simulink model "my_dom_model"  (R2018a)
settings: Solver=VariableStepAuto  StartTime=0.0  StopTime=10000  RelTol=1e-3
values from neighbouring files (symbols this model uses):
  c_p = 1000    [leveled_NL.m]    (also in leveled_state_space.m; leveled_transmitancja.m; my_dom.m; my_dom_state_space_script.m)
  C_vp = c_p*ro_p*V_p    (= 120000)    [leveled_NL.m]    (also in leveled_state_space.m; leveled_transmitancja.m; my_dom.m; my_dom_state_space_script.m)
  C_vw = c_p*ro_p*V_w    (= 1200000)    [leveled_NL.m]    (also in leveled_state_space.m; leveled_transmitancja.m; my_dom.m; my_dom_state_space_script.m)
  d_f_p = 0.2    [leveled_NL.m]    (also in leveled_state_space.m = 0; leveled_transmitancja.m = 0; my_dom.m; my_dom_state_space_script.m = 0)
  d_T_z = 0    [leveled_NL.m]    (also in leveled_state_space.m; leveled_transmitancja.m; my_dom.m; my_dom_state_space_script.m)
  d_T_zew = 0    [leveled_NL.m]    (also in leveled_state_space.m = 2; leveled_transmitancja.m = 2; my_dom.m; my_dom_state_space_script.m = 5)
  f_p1 = f_pN-0.35    (= 0.65)    [leveled_NL.m]    (also in leveled_state_space.m = 1; leveled_transmitancja.m = 1; my_dom.m = 1.25; my_dom_statyczne.m = 0.1:0.1:25)
  K_1 = K_matrix(1,1)    [leveled_NL.m]    (also in leveled_state_space.m; leveled_transmitancja.m; my_dom.m; my_dom_state_space_script.m)
  K_p = p*K_w    [leveled_NL.m]    (also in leveled_state_space.m; leveled_transmitancja.m; my_dom.m; my_dom_state_space_script.m)
  K_w = K_matrix(2,1)    [leveled_NL.m]    (also in leveled_state_space.m; leveled_transmitancja.m; my_dom.m; my_dom_state_space_script.m)
  ro_p = 1.2    [leveled_NL.m]    (also in leveled_state_space.m; leveled_transmitancja.m; my_dom.m; my_dom_state_space_script.m)
  steptime = 1000    [leveled_NL.m]    (also in leveled_state_space.m; leveled_transmitancja.m; my_dom.m; my_dom_state_space_script.m)
  T_p0 = (K_1*T_wew0+K_p*T_zew1)*M    [leveled_NL.m]    (also in leveled_state_space.m; leveled_transmitancja.m; my_dom.m)
  T_wew0 = (c_p*ro_p*f_p1*T_z1+K_1*K_p*T_zew1*M +K_w*T_zew1)/(c_p*ro_p*f_p1+K_1+K_w-(K_1^2)*M)    [leveled_NL.m]    (also in leveled_state_space.m; leveled_transmitancja.m; my_dom.m)
  T_z1 = T_zN+8    (= 32)    [leveled_NL.m]    (also in leveled_state_space.m = 21; leveled_transmitancja.m = 21; my_dom.m = 29; my_dom_statyczne.m = 24)
  T_zew1 = T_zewN-5    (= -6)    [leveled_NL.m]    (also in leveled_state_space.m = 4; leveled_transmitancja.m = 4; my_dom.m; my_dom_statyczne.m = -1)
settings Model: Creator=johnb  LastModifiedBy=john

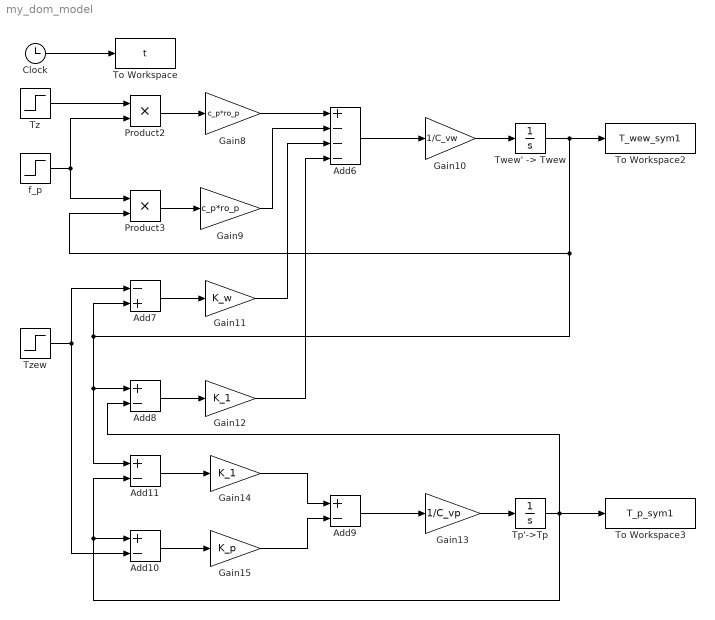
== system my_dom_model ==
  Add{8..11} (4 alike) : Sum  Inputs=+-
  Add6 : Sum  Inputs=+---
  Add7 : Sum  Inputs=-+
  Clock : Clock
  Gain10 : Gain  Gain=1/C_vw
  Gain11 : Gain  Gain=K_w
  Gain12 : Gain  Gain=K_1
  Gain13 : Gain  Gain=1/C_vp
  Gain14 : Gain  Gain=K_1
  Gain15 : Gain  Gain=K_p
  Gain8 : Gain  Gain=c_p*ro_p
  Gain9 : Gain  Gain=c_p*ro_p
  Product2 : Product
  Product3 : Product
  To Workspace : ToWorkspace  VariableName=t  SampleTime=-1
  To Workspace2 : ToWorkspace  VariableName=T_wew_sym1  SampleTime=-1
  To Workspace3 : ToWorkspace  VariableName=T_p_sym1  SampleTime=-1
  Tp'->Tp : Integrator  InitialCondition=T_p0
  "Twew' -> Twew" : Integrator  InitialCondition=T_wew0
  Tz : Step  Time=steptime  Before=T_z1  After=T_z1+d_T_z  SampleTime=0
  "Tzew " : Step  Time=steptime  Before=T_zew1  After=T_zew1+d_T_zew  SampleTime=0
  f_p : Step  Time=steptime  Before=f_p1  After=f_p1+d_f_p  SampleTime=0
  wires:
  Add6/1 -> Gain10/1
  Add11/1 -> Gain14/1
  Add8/1 -> Gain12/1
  Tp'->Tp/1 -> Add8/2, To Workspace3/1, Add11/2, Add10/1
  Add10/1 -> Gain15/1
  Add9/1 -> Gain13/1
  Product3/1 -> Gain9/1
  Gain11/1 -> Add6/3
  Gain10/1 -> "Twew' -> Twew"/1
  Gain15/1 -> Add9/2
  Add7/1 -> Gain11/1
  Gain12/1 -> Add6/4
  Gain14/1 -> Add9/1
  "Tzew "/1 -> Add10/2, Add7/1
  Product2/1 -> Gain8/1
  f_p/1 -> Product2/2, Product3/1
  Gain8/1 -> Add6/1
  Gain9/1 -> Add6/2
  Tz/1 -> Product2/1
  Gain13/1 -> Tp'->Tp/1
  "Twew' -> Twew"/1 -> To Workspace2/1, Add11/1, Add8/1, Add7/2, Product3/2
  Clock/1 -> To Workspace/1
